simulink model "vcpsvdex"  (Simulink 3.00)
settings: Solver=FixedStepDiscrete  StartTime=0.0  StopTime=500.0  FixedStep=Auto  RelTol=1e-3
undefined symbols (not defined in the file or in its folder): m, n
libraries: smxl x8, simulink3 x2
settings Model: LastModifiedBy=giampiero

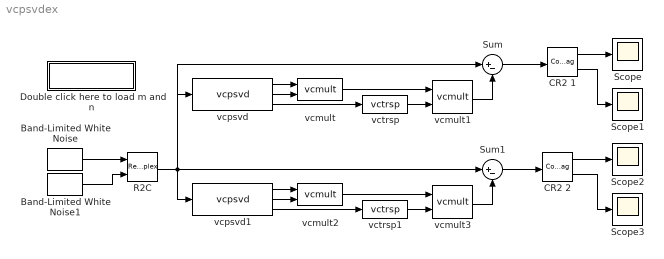
== system vcpsvdex ==
  Band-Limited White Noise : simulink3/Sources/Band-Limited White Noise  Cov=[0.1]*ones(n*m,1)  Ts=0.1  seed=1:(n*m)
  Band-Limited White Noise1 : simulink3/Sources/Band-Limited White Noise  Cov=[0.1]*ones(n*m,1)  Ts=0.1  seed=(n*m)+[1:(n*m)]
  CR2 1 : ComplexToRealImag  Output=RealAndImag
  CR2 2 : ComplexToRealImag  Output=RealAndImag
  Double click here to load m and n : Subsystem
      settings: OpenFcn=m=2;n=3;
      mask Display: disp('Load m and n')
  R2C : RealImagToComplex  Input=RealAndImag  ConstantPart=0
  Scope{,1..3} (4 alike) : Scope
      settings: TimeRange=500  YMin=-1e-014  YMax=1e-014  SaveToWorkspace=off  SaveName=ScopeData
  Sum : Sum  Inputs=|+-  SaturateOnIntegerOverflow=on
  Sum1 : Sum  Inputs=|+-  SaturateOnIntegerOverflow=on
  vcmult : smxl/Complex Matrices/vcmult  d=[n 2*min(m,n) 2*min(m,n)]
  vcmult1 : smxl/Complex Matrices/vcmult  d=[n 2*min(m,n) m]
  vcmult2 : smxl/Complex Matrices/vcmult  d=[m 2*min(m,n) 2*min(m,n)]
  vcmult3 : smxl/Complex Matrices/vcmult  d=[m 2*min(m,n) n]
  vcpsvd : smxl/Complex Matrices/vcpsvd  d=[n m]
  vcpsvd1 : smxl/Complex Matrices/vcpsvd  d=[m n]
  vctrsp : smxl/Complex Matrices/vctrsp  d=[m 2*min(m,n)]  h=on
  vctrsp1 : smxl/Complex Matrices/vctrsp  d=[n 2*min(m,n)]  h=on
  wires:
  vcmult1/1 -> Sum/2
  CR2 1/1 -> Scope/1
  CR2 1/2 -> Scope1/1
  Sum/1 -> CR2 1/1
  vcmult3/1 -> Sum1/2
  Sum1/1 -> CR2 2/1
  vcpsvd1/1 -> vcmult2/1
  vcpsvd1/2 -> vcmult2/2
  CR2 2/1 -> Scope2/1
  CR2 2/2 -> Scope3/1
  vcpsvd/2 -> vcmult/2
  vcpsvd/1 -> vcmult/1
  vcmult/1 -> vcmult1/1
  vctrsp/1 -> vcmult1/2
  vcmult2/1 -> vcmult3/1
  vctrsp1/1 -> vcmult3/2
  vcpsvd1/3 -> vctrsp1/1
  vcpsvd/3 -> vctrsp/1
  R2C/1 -> vcpsvd/1, Sum/1, Sum1/1, vcpsvd1/1
  Band-Limited White Noise/1 -> R2C/1
  Band-Limited White Noise1/1 -> R2C/2

== system vcpsvdex/Double click here to load m and n ==
